simulink model "manual"  (R2019b)
settings: Solver=ode4  StartTime=0.0  StopTime=3000  FixedStep=1  RelTol=1e-3
libraries: simulink_extras x2, simulink x1
settings Model: Creator=shao  LastModifiedBy=shao

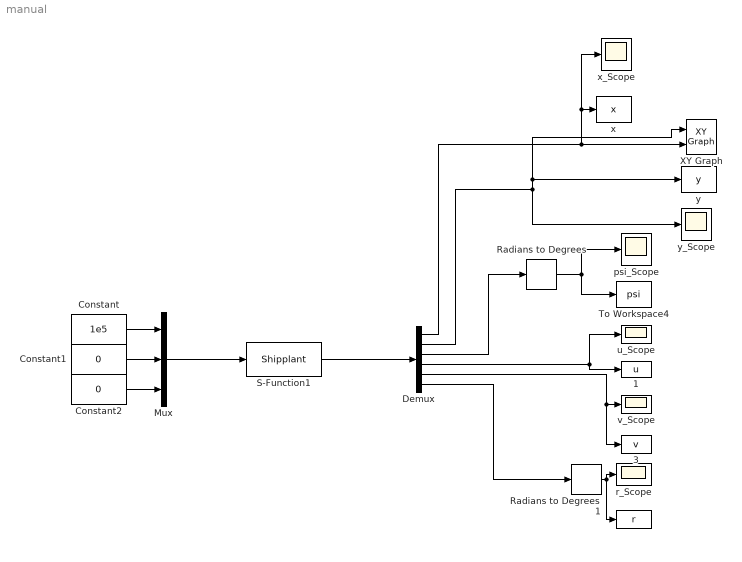
== system manual ==
  " " : ToWorkspace  VariableName=r  SampleTime=-1
  " 1" : ToWorkspace  VariableName=u  SampleTime=-1
  " 3" : ToWorkspace  VariableName=v  SampleTime=-1
  Constant : Constant  Value=1e5
  Constant1 : Constant  Value=0
  Constant2 : Constant  Value=0
  Demux : Demux  Outputs=6
  Mux : Mux  Inputs=3
  "Radians to Degrees  " : simulink_extras/Transformations/Radians to Degrees
  Radians to Degrees  1 : simulink_extras/Transformations/Radians to Degrees
  S-Function1 : S-Function  FunctionName=Shipplant  SFunctionDeploymentMode=off  EnableBusSupport=off
  To Workspace4 : ToWorkspace  VariableName=psi  SampleTime=-1
  XY Graph : simulink/Sinks/XY Graph  xmin=-1  xmax=6  ymin=-1  ymax=5  st=-1
  psi_Scope : Scope
  r_Scope : Scope
  u_Scope : Scope
  v_Scope : Scope
  x : ToWorkspace  VariableName=x  SampleTime=-1
  x_Scope : Scope
  y : ToWorkspace  VariableName=y  SampleTime=-1
  y_Scope : Scope
  wires:
  Mux/1 -> S-Function1/1
  Constant/1 -> Mux/1
  Constant1/1 -> Mux/2
  Constant2/1 -> Mux/3
  S-Function1/1 -> Demux/1
  Demux/1 -> x_Scope/1, x/1, XY Graph/2
  Demux/2 -> XY Graph/1, y/1, y_Scope/1
  Demux/5 -> " 3"/1, v_Scope/1
  Demux/4 -> u_Scope/1, " 1"/1
  Radians to Degrees  1/1 -> " "/1, r_Scope/1
  "Radians to Degrees  "/1 -> To Workspace4/1, psi_Scope/1
  Demux/3 -> "Radians to Degrees  "/1
  Demux/6 -> Radians to Degrees  1/1
